simulink model "SimulinkDroneWorld_automatic"  (R2020a)
settings: Solver=VariableStepAuto  StartTime=0.0  StopTime=76  RelTol=1e-3
libraries: vrlib x1
settings Model: Creator=rjvar  LastModifiedBy=rjvar

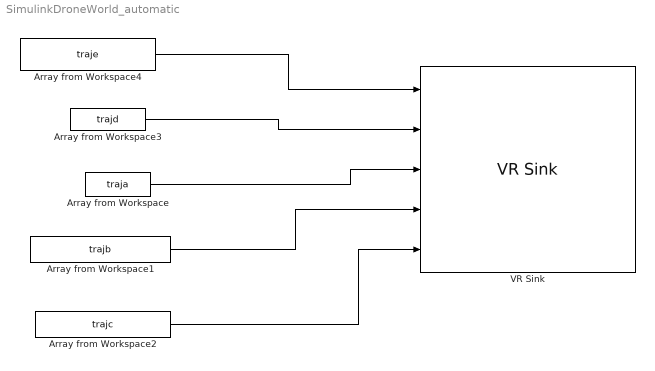
== system SimulinkDroneWorld_automatic ==
  Array from Workspace : FromWorkspace  VariableName=traja
  Array from Workspace1 : FromWorkspace  VariableName=trajb
  Array from Workspace2 : FromWorkspace  VariableName=trajc
  Array from Workspace3 : FromWorkspace  VariableName=trajd  OutDataTypeStr=double
  Array from Workspace4 : FromWorkspace  VariableName=traje
  VR Sink : vrlib/VR Sink  InstantiateOnLoad=on  SampleTime=0.02  ViewEnable=on  RemoteChange=off  RemoteView=off  FieldsWritten=View.rotation.4.1.1.double#View.translation.3.1.1.double#Drone1.translation.3.1.1.double#Drone2.translation.3.1.1.double#Drone3.translation.3.1.1.double  WorldFileName=C:\Users\rjvar\Dropbox\My PC (LAPTOP-HLU14FS6)\Desktop\CPS-Project-main\3-D Simulation\World-Model\Disaster_Prob.x3d  AutoView=off  VideoDimensions=[]  AllowVariableSize=off  FigureProperties="{'Position', 'Name', 'Viewpoint', 'CameraBound', 'CameraDirection', 'CameraPosition', 'CameraUpVector', 'ZoomFactor', 'Antialiasing', 'Headlight', 'Lighting', 'NavPanel', 'Sound', 'StatusBar', 'Stereo3D', 'Stereo3DCameraOffset', 'Stereo3DHIT', 'ToolBar', 'Textures', 'Transparency', 'Triad', 'Wireframe', 'NavZones', 'NavMode', 'NavSpeed', 'CaptureFileFormat', 'CaptureFileName', 'Record2DCompressMethod', 'Record2DCompressQuality', 'Record2D', 'Record2DFileName', 'Record2DFPS'; [1.0000000000000000e+00   7.4199999999999932e+01   1.5360000000000000e+03   6.9880000000000007e+02], '', '_untitled_1', 'on', [0.0000000000000000e+00   0.0000000000000000e+00  -1.0000000000000000e+00], [0.0000000000000000e+00   0.0000000000000000e+00   0.0000000000000000e+00], [0.0000000000000000e+00   1.0000000000000000e+00   0.0000000000000000e+00], [1.0000000000000000e+00], 'on', 'on', 'on', 'halfbar', 'on', 'on', 'off', [1.0000000149011612e-01], [0.0000000000000000e+00], 'on', 'on', 'on', 'none', 'off', 'off', 'fly', 'normal', 'tif', '%f_anim_%n.tif', 'auto', [2.1000000000000000e+01], 'on', 'C:\\Users\\rjvar\\Dropbox\\My PC (LAPTOP-HLU14FS6)\\Desktop\\Drone Motion without Intersource.avi', 'auto'}"
  wires:
  Array from Workspace/1 -> VR Sink/3
  Array from Workspace1/1 -> VR Sink/4
  Array from Workspace2/1 -> VR Sink/5
  Array from Workspace3/1 -> VR Sink/2
  Array from Workspace4/1 -> VR Sink/1
